simulink model "complex_motor"  (R2015a)
settings: Solver=ode3  StartTime=0.0  StopTime=5  FixedStep=0.001  RelTol=1e-3
settings Model: Creator=LAB425  LastModifiedBy=LAB425

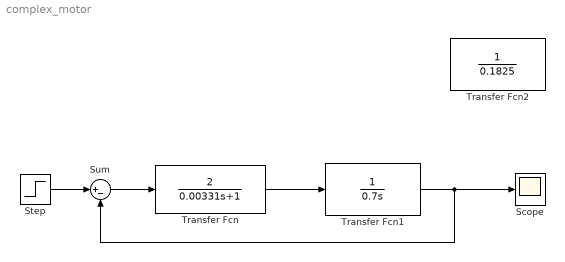
== system complex_motor ==
  Scope : Scope
  Step : Step  Time=0  SampleTime=0
  Sum : Sum  Inputs=|+-
  Transfer Fcn : TransferFcn  Numerator=[2]  Denominator=[0.00331 1]
  Transfer Fcn1 : TransferFcn  Denominator=[0.7 0]
  Transfer Fcn2 : TransferFcn  Denominator=[0.1825]
  wires:
  Transfer Fcn1/1 -> Scope/1, Sum/2
  Transfer Fcn/1 -> Transfer Fcn1/1
  Step/1 -> Sum/1
  Sum/1 -> Transfer Fcn/1
